simulink model "SeesawModel"  (R2015a)
settings: Solver=ode3  StartTime=0.0  StopTime=2  FixedStep=0.01  RelTol=1e-3
values from neighbouring files (symbols this model uses):
  b = 1    [SeesawModel_parameters.m]
  g = 9.8    [SeesawModel_parameters.m]
  J = 1    [SeesawModel_parameters.m]
  K = 1    [SeesawModel_parameters.m]
  L = 1    [SeesawModel_parameters.m]
  md = 1    [SeesawModel_parameters.m]
  mp = 1    [SeesawModel_parameters.m]
  mr = 1    [SeesawModel_parameters.m]
  R = 1    [SeesawModel_parameters.m]
  rwheel = 1    [SeesawModel_parameters.m]
  testStep = 1    [SeesawModel_parameters.m]
  x2 = 1    [SeesawModel_parameters.m]
settings Model: Creator=Administrator  LastModifiedBy=Administrator

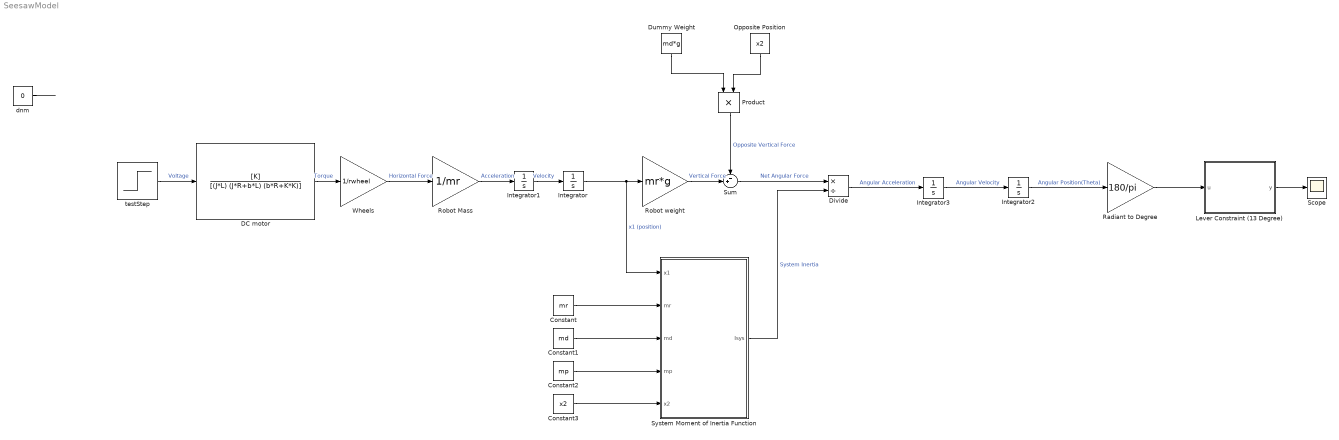
== system SeesawModel ==
  Constant : Constant  Value=mr
  Constant1 : Constant  Value=md
  Constant2 : Constant  Value=mp
  Constant3 : Constant  Value=x2
  DC motor : TransferFcn  Numerator=[K]  Denominator=[(J*L) (J*R+b*L) (b*R+K*K)]
  Divide : Product  Inputs=*/
  Dummy Weight : Constant  Value=md*g
  Integrator : Integrator
  Integrator1 : Integrator
  Integrator2 : Integrator
  Integrator3 : Integrator  UpperSaturationLimit=100
  Lever Constraint (13 Degree) : MATLAB Function  TreatAsAtomicUnit=on
  Opposite Position : Constant  Value=x2
  Product : Product
  Radiant to Degree : Gain  Gain=180/pi
  Robot Mass : Gain  Gain=1/mr
  Robot weight : Gain  Gain=mr*g
  Scope : Scope
  Sum : Sum  Inputs=-+|
  System Moment of Inertia Function : MATLAB Function  TreatAsAtomicUnit=on
  Wheels : Gain  Gain=1/rwheel
  dnm : Constant  Value=0
  testStep : Step  After=testStep  SampleTime=0
  wires:
  testStep/1 -> DC motor/1  "Voltage"
  DC motor/1 -> Wheels/1  "Torque"
  Wheels/1 -> Robot Mass/1  "Horizontal Force"
  Robot Mass/1 -> Integrator1/1  "Acceleration"
  Integrator1/1 -> Integrator/1  "Velocity"
  Integrator/1 -> System Moment of Inertia Function/1(x1), Robot weight/1  "x1 (position)"
  Dummy Weight/1 -> Product/1
  Opposite Position/1 -> Product/2
  Product/1 -> Sum/1  "Opposite Vertical Force"
  Robot weight/1 -> Sum/2  "Vertical Force"
  Sum/1 -> Divide/1  "Net Angular Force"
  Divide/1 -> Integrator3/1  "Angular Acceleration"
  Integrator3/1 -> Integrator2/1  "Angular Velocity"
  Integrator2/1 -> Radiant to Degree/1  "Angular Position(Theta)"
  System Moment of Inertia Function/1(Isys) -> Divide/2  "System Inertia"
  Constant/1 -> System Moment of Inertia Function/2(mr)
  Constant3/1 -> System Moment of Inertia Function/5(x2)
  Constant2/1 -> System Moment of Inertia Function/4(mp)
  Constant1/1 -> System Moment of Inertia Function/3(md)
  Lever Constraint (13 Degree)/1(y) -> Scope/1
  Radiant to Degree/1 -> Lever Constraint (13 Degree)/1(u)
  dnm/1 -> ?

== matlab function SeesawModel/Lever Constraint (13 Degree) ==
  data: u input; y output
function y = leverConstraint(u)
if u>=13
    y=13;
elseif u<=-13
    y=-13;
else
    y=u;
end

== matlab function SeesawModel/System Moment of Inertia Function ==
  data: x1 input; Isys output; mr input; md input; mp input; x2 input
function Isys = Inertia(x1, mr, md, mp, x2)
M=mr+md+mp;
Mmasses=mr+md;
Isys=M*((Mmasses*((mr*x1+md*x2)/Mmasses))/M)^2;
